simulink model "SimulinkFinal"  (R2023b)
settings: Solver=FixedStepAuto  StartTime=0.0  StopTime=inf  FixedStep=0.01  RelTol=1e-3
StopFcn:
  | % Generate a unique filename based on the current date and time
  | timestamp = datestr(now, 'yyyy-mm-dd_HH-MM-SS');
  | filename = ['simulation_logs_' timestamp '.mat'];
  | 
  | % Check if 'out' variable (SimulationOutput) exists
  | if exist('out', 'var')
  |     % Extract logsout from the simulation output object
  |     logsout = out.logsout;
  | 
  |     % Save the logsout variable to a .mat file
  |     save(filename, 'logsout');
  | else
  |     warning('Simulation output not found. No data saved.');
  | end
model workspace (MAT data in the model file):
  SL_ROS_VariableLengthArrays_MaxSizes.CommonInfo.ArrayTruncateAction = 'EmitWarning'
  SL_ROS_VariableLengthArrays_MaxSizes.MsgTypeMap = containers.Map
  SL_ROS_VariableLengthArrays_MaxSizes.MsgTypeMap.serialization.keys = {'sensor_msgs/Image', 'sensor_msgs/PointCloud2'}
  SL_ROS_VariableLengthArrays_MaxSizes.MsgTypeMap.serialization.values{1}(1).PropertyName = 'data'
  SL_ROS_VariableLengthArrays_MaxSizes.MsgTypeMap.serialization.values{1}(1).DataType = 'uint8'
  SL_ROS_VariableLengthArrays_MaxSizes.MsgTypeMap.serialization.values{1}(1).MaxLength = 1920000
  SL_ROS_VariableLengthArrays_MaxSizes.MsgTypeMap.serialization.values{1}(2).PropertyName = 'encoding'
  SL_ROS_VariableLengthArrays_MaxSizes.MsgTypeMap.serialization.values{1}(2).DataType = 'uint8'
  SL_ROS_VariableLengthArrays_MaxSizes.MsgTypeMap.serialization.values{1}(2).MaxLength = 128
  SL_ROS_VariableLengthArrays_MaxSizes.MsgTypeMap.serialization.values{2}(1).PropertyName = 'data'
  SL_ROS_VariableLengthArrays_MaxSizes.MsgTypeMap.serialization.values{2}(1).DataType = 'uint8'
  SL_ROS_VariableLengthArrays_MaxSizes.MsgTypeMap.serialization.values{2}(1).MaxLength = 390000
  SL_ROS_VariableLengthArrays_MaxSizes.MsgTypeMap.serialization.values{2}(2).PropertyName = 'fields'
  SL_ROS_VariableLengthArrays_MaxSizes.MsgTypeMap.serialization.values{2}(2).DataType = 'sensor_msgs/PointField'
  SL_ROS_VariableLengthArrays_MaxSizes.MsgTypeMap.serialization.values{2}(2).MaxLength = 16
  SL_ROS_VariableLengthArrays_MaxSizes.MsgTypeMap.serialization.uniformity = 0
  SL_ROS_VariableLengthArrays_MaxSizes.MsgTypeMap.serialization.keyType = 'char'
  SL_ROS_VariableLengthArrays_MaxSizes.MsgTypeMap.serialization.valueType = 'any'
undefined symbols (not defined in the file or in its folder): brake, reverse, steer, throttle
libraries: ros2lib x7, slpidlib x1
settings Model: Creator=pruthvi  LastModifiedBy=pruthvi
settings OptimizationCC: EnhancedBackFolding=on  PassReuseOutputArgsAs=Individual arguments  ZeroExternalMemoryAtStartup=off  ZeroInternalMemoryAtStartup=off  MaxStackSize=64  OptimizeBlockOrder=speed  DifferentSizesBufferReuse=on  OptimizationCustomize=off  EfficientTunableParamExpr=on
settings DebuggingCC: ParameterPrecisionLossMsg=none  ParameterTunabilityLossMsg=error
settings HardwareCC: UseEmbeddedCoderFeatures=off
settings SFSimCC: MATLABDynamicMemAlloc=off
settings RTWCC: Description=Embedded Coder  SystemTargetFile=ert.tlc  HardwareBoard=Robot Operating System 2 (ROS 2)  TLCOptions="-aInlineSetEventsForThisBaseRateFcn=TLC_FALSE -aSuppressMultiTaskScheduler=TLC_FALSE  -aRateBasedStepFcn=0"  TemplateMakefile=ert_default_tmf  Toolchain=Colcon Tools  TargetLang=C++
settings CodeAppCC: ForceParamTrailComments=on  IgnoreCustomStorageClasses=off  OperatorAnnotations=on  SimulinkDataObjDesc=on  SFDataObjDesc=on  InsertBlockDesc=on
settings ERTTargetCC: CodeInterfacePackaging=C++ class  SupportNonInlinedSFcns=on  RootIOFormat=Structure reference

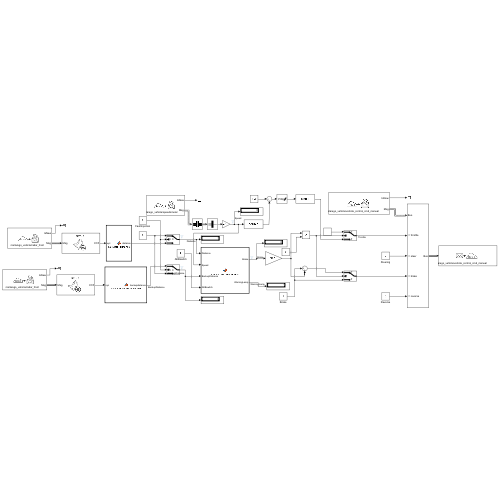
[thumbnail: Simulink's stored preview of the top-level diagram]
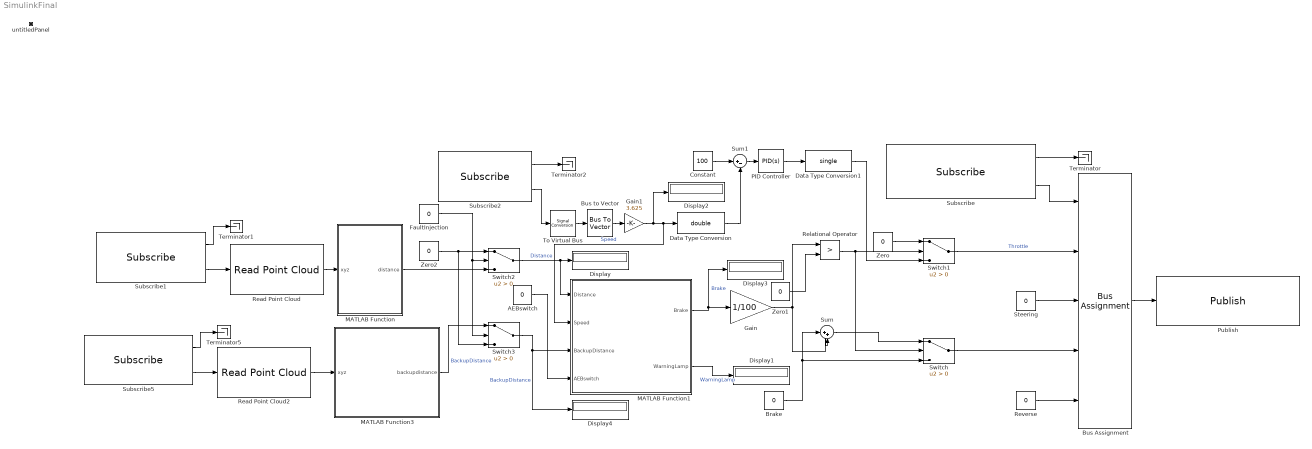
== system SimulinkFinal ==
  AEBswitch : Constant  Value=0  OutDataTypeStr=uint8
  Brake : Constant  Value=0  OutDataTypeStr=single
  Bus Assignment : BusAssignment  AssignedSignals=throttle,steer,brake,reverse
  Bus to Vector : BusToVector
  Constant : Constant  Value=100  OutDataTypeStr=double
  Data Type Conversion : DataTypeConversion  OutDataTypeStr=double  RndMeth=Round  SaturateOnIntegerOverflow=off
  Data Type Conversion1 : DataTypeConversion  OutDataTypeStr=single  RndMeth=Floor
  Display{,1..4} (5 alike) : Display
  FaultInjection : Constant  Value=0
  Gain : Gain  Gain=1/100  OutDataTypeStr=single  RndMeth=Simplest
  Gain1 : Gain  Gain=3.625  OutDataTypeStr=uint8  RndMeth=Round  SaturateOnIntegerOverflow=on
  MATLAB Function : MATLAB Function  TreatAsAtomicUnit=on  SystemSampleTime=0.01
  MATLAB Function1 : MATLAB Function  TreatAsAtomicUnit=on  SystemSampleTime=0.01
  MATLAB Function3 : MATLAB Function  TreatAsAtomicUnit=on  SystemSampleTime=0.01
  PID Controller : slpidlib/PID Controller  Controller=PID  Form=Parallel  TimeDomain=Continuous-time  UseExternalTs=off  SampleTime=-1  IntegratorMethod=Forward Euler  FilterMethod=Forward Euler  ControllerParametersSource=internal  P=0.2  I=0.03  UseKiTs=off  D=0.2  N=100  UseFilter=on  TunerSelectOption=Transfer Function Based (PID Tuner App)  InitialConditionSource=internal  InitialConditionForIntegrator=0  InitialConditionForFilter=0  DifferentiatorICPrevScaledInput=0  ExternalReset=none  TrackingMode=off  Kt=1  LimitOutput=on  SatLimitsSource=internal  UpperSaturationLimit=1  LowerSaturationLimit=0  LinearizeAsGain=on  AntiWindupMode=clamping  Kb=1  LimitIntegrator=on  UpperIntegratorSaturationLimit=1  LowerIntegratorSaturationLimit=0  POutMin=[]  POutMax=[]  IOutMin=[]  IOutMax=[]  DOutMin=[]  DOutMax=[]  NOutMin=[]  NOutMax=[]  SumOutMin=[]  SumOutMax=[]  SaturationOutMin=[]  SaturationOutMax=[]  PParamMin=[]  PParamMax=[]  IParamMin=[]  IParamMax=[]  DParamMin=[]  DParamMax=[]  NParamMin=[]  NParamMax=[]  KbParamMin=[]  KbParamMax=[]  KtParamMin=[]  KtParamMax=[]  KbOutMin=[]  KbOutMax=[]  KtOutMin=[]  KtOutMax=[]  IntegratorOutMin=[]  IntegratorOutMax=[]  FilterOutMin=[]  FilterOutMax=[]  SumI1OutMin=[]  SumI1OutMax=[]  SumI2OutMin=[]  SumI2OutMax=[]  SumI3OutMin=[]  SumI3OutMax=[]  SumI4OutMin=[]  SumI4OutMax=[]  SumDOutMin=[]  SumDOutMax=[]  DifferentiatorOutMin=[]  DifferentiatorOutMax=[]  FilterDiffOutCoefMin=[]  FilterDiffOutCoefMax=[]  ReciprocalOutMin=[]  ReciprocalOutMax=[]  SumDenOutMin=[]  SumDenOutMax=[]  SumNumOutMin=[]  SumNumOutMax=[]  DivideOutMin=[]  DivideOutMax=[]  UdiffTsProdOutMin=[]  UdiffTsProdOutMax=[]  NTsProdOutMin=[]  NTsProdOutMax=[]  UintegralTsProdOutMin=[]  UintegralTsProdOutMax=[]  UngainTsProdOutMin=[]  UngainTsProdOutMax=[]  ClampingZeroOutDataTypeStr=Inherit: Inherit via back propagation  ClampingZeroOutMin=[]  ClampingZeroOutMax=[]  FilterDenConstantOutDataTypeStr=Inherit: Inherit via back propagation  FilterDenConstantOutMin=[]  FilterDenConstantOutMax=[]  PCopyOutDataTypeStr=Inherit: Inherit via back propagation  PCopyOutMin=[]  PCopyOutMax=[]  NCopyOutDataTypeStr=Inherit: Inherit via back propagation  NCopyOutMin=[]  NCopyOutMax=[]  IntegratorContinuousStateAttributes=''  IntegratorStateMustResolveToSignalObject=off  IntegratorRTWStateStorageClass=Auto  FilterContinuousStateAttributes=''  FilterStateMustResolveToSignalObject=off  FilterRTWStateStorageClass=Auto  ParallelPVariant=InternalParameters  IdealPVariant=Disabled  IVariant=InternalParameters  DVariant=InternalParameters  IntegratorVariant=Continuous  SatVariant=Enabled  AWVariant=ContClampingParallel  PCopyVariant=Disabled  TRVariant=Disabled  FdbkBlocksVariant=Forward  IdealPFdbkVariant=Disabled  SatFdbkVariant=Disabled  DerivativeFilterVariant=ContFilter  NVariant=InternalParameters  NCopyVariant=Disabled  FilterICVariant=InternalICsFilter  IntegratorICVariant=InternalICs  ExternalResetVariant=Disabled  TRSumVariant=Passthrough  SumFdbkVariant=Disabled  SumVariant=Sum_PID  TsampFilterVariant=InternalTs  TsampNgainVariant=Passthrough  TsampIntegralVariant=Disabled_SignalSpec  ExternalSaturationOutDataTypeStr=Inherit: Same as second input
  Publish : ros2lib/Publish  topicSource=Select from ROS network  topic=/carla/ego_vehicle/vehicle_control_cmd_manual  messageType=carla_msgs/CarlaEgoVehicleControl  QOSHistory=Keep last  QOSDepth=1  QOSReliability=Reliable  QOSDurability=Volatile
  Read Point Cloud : ros2lib/Read Point Cloud  MaximumPointCloudSize=[1, 8254]  PreserveStructure=off  ShowRGBOutput=off  ShowIntensityOutput=off  ShowErrorCodeOutput=off  VariableSizeOutputs=off
  Read Point Cloud2 : ros2lib/Read Point Cloud  MaximumPointCloudSize=[1, 8254]  PreserveStructure=off  ShowRGBOutput=off  ShowIntensityOutput=off  ShowErrorCodeOutput=off  VariableSizeOutputs=off
  Relational Operator : RelationalOperator  Operator=>  OutDataTypeStr=boolean  RndMeth=Simplest  InputSameDT=off
  Reverse : Constant  Value=0  OutDataTypeStr=boolean
  Steering : Constant  Value=0  OutDataTypeStr=single
  Subscribe : ros2lib/Subscribe  topicSource=Select from ROS network  topic=/carla/ego_vehicle/vehicle_control_cmd_manual  messageType=carla_msgs/CarlaEgoVehicleControl  sampleTime=-1  QOSHistory=Keep last  QOSDepth=1  QOSReliability=Reliable  QOSDurability=Volatile
  Subscribe1 : ros2lib/Subscribe  topicSource=Select from ROS network  topic=/carla/ego_vehicle/radar_front  messageType=sensor_msgs/PointCloud2  sampleTime=0.2  QOSHistory=Keep last  QOSDepth=1  QOSReliability=Reliable  QOSDurability=Volatile
  Subscribe2 : ros2lib/Subscribe  topicSource=Select from ROS network  topic=/carla/ego_vehicle/speedometer  messageType=std_msgs/Float32  sampleTime=-1  QOSHistory=Keep last  QOSDepth=1  QOSReliability=Reliable  QOSDurability=Volatile
  Subscribe5 : ros2lib/Subscribe  topicSource=Select from ROS network  topic=/carla/ego_vehicle/radar_front  messageType=sensor_msgs/PointCloud2  sampleTime=0.2  QOSHistory=Keep last  QOSDepth=1  QOSReliability=Reliable  QOSDurability=Volatile
  Sum : Sum  Inputs=|++
  Sum1 : Sum  Inputs=|+-
  Switch{,1..3} (4 alike) : Switch  Criteria=u2 > Threshold  SaturateOnIntegerOverflow=off  InputSameDT=off
  Terminator{,1..2,5} (4 alike) : Terminator
  To Virtual Bus : SignalConversion  ConversionOutput=Virtual bus  OverrideOpt=off
  Zero : Constant  Value=0  OutDataTypeStr=Inherit: Inherit via back propagation
  Zero1 : Constant  Value=0  OutDataTypeStr=Inherit: Inherit via back propagation
  Zero2 : Constant  Value=0  OutDataTypeStr=Inherit: Inherit via back propagation
  untitledPanel : Subsystem  Tag=HiddenForWebPanel  IsWebBlockPanel=on
  wires:
  Subscribe2/1 -> Terminator2/1
  Subscribe5/1 -> Terminator5/1
  Constant/1 -> Sum1/1
  Subscribe1/2 -> Read Point Cloud/1
  Data Type Conversion1/1 -> Switch1/3
  To Virtual Bus/1 -> Bus to Vector/1
  Subscribe1/1 -> Terminator1/1
  Zero/1 -> Switch1/1
  Subscribe2/2 -> To Virtual Bus/1
  MATLAB Function/1(distance) -> Switch2/3
  Bus to Vector/1 -> Gain1/1
  Data Type Conversion/1 -> Sum1/2
  Subscribe5/2 -> Read Point Cloud2/1
  Read Point Cloud/1 -> MATLAB Function/1(xyz)
  Zero1/1 -> Relational Operator/2
  Read Point Cloud2/1 -> MATLAB Function3/1(xyz)
  Reverse/1 -> Bus Assignment/5
  Gain1/1 -> Display2/1, MATLAB Function1/2(Speed), Data Type Conversion/1  "Speed"
  Sum1/1 -> PID Controller/1
  FaultInjection/1 -> Switch3/2, Switch2/2
  Steering/1 -> Bus Assignment/3
  Zero2/1 -> Switch2/1, Switch3/3
  MATLAB Function3/1(backupdistance) -> Switch3/1  "BackupDistance"
  Switch2/1 -> MATLAB Function1/1(Distance), Display/1  "Distance"
  MATLAB Function1/1(Brake) -> Display3/1, Gain/1  "Brake"
  AEBswitch/1 -> MATLAB Function1/4(AEBswitch)
  PID Controller/1 -> Data Type Conversion1/1
  Switch3/1 -> MATLAB Function1/3(BackupDistance), Display4/1  "BackupDistance"
  Switch1/1 -> Bus Assignment/2  "Throttle"
  Relational Operator/1 -> Switch/2, Switch1/2
  MATLAB Function1/2(WarningLamp) -> Display1/1  "WarningLamp"
  Gain/1 -> Sum/2, Relational Operator/1
  Brake/1 -> Sum/1, Switch/3
  Sum/1 -> Switch/1
  Subscribe/1 -> Terminator/1
  Subscribe/2 -> Bus Assignment/1
  Switch/1 -> Bus Assignment/4
  Bus Assignment/1 -> Publish/1

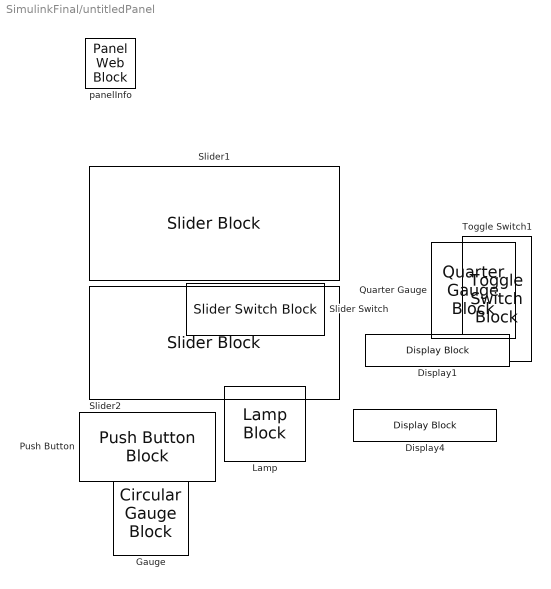
== system SimulinkFinal/untitledPanel ==
  Display1 : DisplayBlock  Tag=HiddenForWebPanel  PanelInfo="{\"addnFilesFolder\":\"\",\"height\":59,\"includeDebugPackages\":false,\"left\":281,\"outputFolder\":\"\",\"panelId\":\"panelId-4ec24f18-4b2b-4da9-8655-6245c59e87f1\",\"popoutMode\":\"\",\"standaloneTitle\":\"\",\"top\":316,\"type\":\"panelChild\",\"version\":\"2019b\",\"width\":174,\"zIndex\":1500038}"  Transparency=1
  Display4 : DisplayBlock  Tag=HiddenForWebPanel  PanelInfo="{\"addnFilesFolder\":\"\",\"height\":60,\"includeDebugPackages\":false,\"left\":283,\"outputFolder\":\"\",\"panelId\":\"panelId-4ec24f18-4b2b-4da9-8655-6245c59e87f1\",\"popoutMode\":\"\",\"standaloneTitle\":\"\",\"top\":386,\"type\":\"panelChild\",\"version\":\"2019b\",\"width\":169,\"zIndex\":1500040}"  Transparency=1
  Gauge : CircularGaugeBlock  Tag=HiddenForWebPanel  PanelInfo="{\"addnFilesFolder\":\"\",\"height\":153,\"includeDebugPackages\":false,\"left\":274,\"outputFolder\":\"\",\"panelId\":\"panelId-4ec24f18-4b2b-4da9-8655-6245c59e87f1\",\"popoutMode\":\"\",\"standaloneTitle\":\"\",\"top\":23,\"type\":\"panelChild\",\"version\":\"2019b\",\"width\":194,\"zIndex\":1500022}"  TickInterval=10
  Lamp : LampBlock  Tag=HiddenForWebPanel  PanelInfo="{\"addnFilesFolder\":\"\",\"height\":65,\"includeDebugPackages\":false,\"left\":178,\"outputFolder\":\"\",\"panelId\":\"panelId-4ec24f18-4b2b-4da9-8655-6245c59e87f1\",\"popoutMode\":\"\",\"standaloneTitle\":\"\",\"top\":365,\"type\":\"panelChild\",\"version\":\"2019b\",\"width\":96,\"zIndex\":1500042}"
  Push Button : PushButtonBlock  Tag=HiddenForWebPanel  PanelInfo="{\"addnFilesFolder\":\"\",\"height\":87,\"includeDebugPackages\":false,\"left\":19,\"outputFolder\":\"\",\"panelId\":\"panelId-4ec24f18-4b2b-4da9-8655-6245c59e87f1\",\"popoutMode\":\"\",\"standaloneTitle\":\"\",\"top\":361,\"type\":\"panelChild\",\"version\":\"2019b\",\"width\":151,\"zIndex\":1500044}"  LabelPosition=Top  ButtonText=SensorFailure  ButtonType=Latch  Icon=CheckEngine2  IconColor=On  OffValue=0.000000
  Quarter Gauge : QuarterGaugeBlock  Tag=HiddenForWebPanel  PanelInfo="{\"addnFilesFolder\":\"\",\"height\":121,\"includeDebugPackages\":false,\"left\":283,\"outputFolder\":\"\",\"panelId\":\"panelId-4ec24f18-4b2b-4da9-8655-6245c59e87f1\",\"popoutMode\":\"\",\"standaloneTitle\":\"\",\"top\":183,\"type\":\"panelChild\",\"version\":\"2019b\",\"width\":168,\"zIndex\":1500024}"  TickInterval=25
  Slider Switch : SliderSwitchBlock  Tag=HiddenForWebPanel  PanelInfo="{\"addnFilesFolder\":\"\",\"height\":54,\"includeDebugPackages\":false,\"left\":105,\"outputFolder\":\"\",\"panelId\":\"panelId-4ec24f18-4b2b-4da9-8655-6245c59e87f1\",\"popoutMode\":\"\",\"standaloneTitle\":\"\",\"top\":268,\"type\":\"panelChild\",\"version\":\"2019b\",\"width\":146,\"zIndex\":1500036}"
      settings: Values={{'Off', 'On'}, [0 1]}
  Slider1 : SliderBlock  Tag=HiddenForWebPanel  PanelInfo="{\"addnFilesFolder\":\"\",\"height\":114,\"includeDebugPackages\":false,\"left\":15,\"outputFolder\":\"\",\"panelId\":\"panelId-4ec24f18-4b2b-4da9-8655-6245c59e87f1\",\"popoutMode\":\"\",\"standaloneTitle\":\"\",\"top\":18,\"type\":\"panelChild\",\"version\":\"2019b\",\"width\":250,\"zIndex\":1500018}"  ScaleMin=-1  ScaleMax=1  TickInterval=1
  Slider2 : SliderBlock  Tag=HiddenForWebPanel  PanelInfo="{\"addnFilesFolder\":\"\",\"height\":113,\"includeDebugPackages\":false,\"left\":15,\"outputFolder\":\"\",\"panelId\":\"panelId-4ec24f18-4b2b-4da9-8655-6245c59e87f1\",\"popoutMode\":\"\",\"standaloneTitle\":\"\",\"top\":138,\"type\":\"panelChild\",\"version\":\"2019b\",\"width\":250,\"zIndex\":1500010}"  ScaleMax=1  TickInterval=0.5
  Toggle Switch1 : ToggleSwitchBlock  Tag=HiddenForWebPanel  PanelInfo="{\"addnFilesFolder\":\"\",\"height\":96,\"includeDebugPackages\":false,\"left\":19,\"outputFolder\":\"\",\"panelId\":\"panelId-4ec24f18-4b2b-4da9-8655-6245c59e87f1\",\"popoutMode\":\"\",\"standaloneTitle\":\"\",\"top\":258,\"type\":\"panelChild\",\"version\":\"2019b\",\"width\":50,\"zIndex\":1500008}"
      settings: Values={{'Off', 'On'}, [0 1]}
  panelInfo : PanelWebBlock  Tag=HiddenForWebPanel  PanelInfo="{\"addnFilesFolder\":\"\",\"compacted\":false,\"height\":465,\"includeDebugPackages\":false,\"isActiveTab\":true,\"left\":17,\"name\":\"Panel\",\"outputFolder\":\"\",\"panelId\":\"panelId-4ec24f18-4b2b-4da9-8655-6245c59e87f1\",\"popoutMode\":\"\",\"standaloneTitle\":\"\",\"tabIndex\":0,\"tabbedSetId\":\"tabbedSet3834338684\",\"top\":33,\"type\":\"panel\",\"version\":\"2019b\",\"visible\":true,\"width\":474,\"zIndex\":1500002}"

== matlab function SimulinkFinal/MATLAB Function1 ==
  data: Distance input; Speed input; BackupDistance input; AEBswitch input; Brake output; WarningLamp output
function [Brake, WarningLamp] = emergencyBrakingLogic(Distance, Speed, BackupDistance, AEBswitch)
% EMERGENCYBRAKINGLOGIC Calculate brake intensity based on filtered distance
% Distance: Smoothed distance data (single)
% Speed: Vehicle speed in kmph (uint8)
% BackupDistance: Backup distance input in case primary fails (uint8)
% AEBswitch: Automatic Emergency Braking switch (1 for ON, 0 for OFF)
% Brake: Braking intensity as a value from 0 to 100 (uint8)
% WarningLamp: Warning signal output (1 if primary sensor fails, 0 otherwise)

persistent brake_history brake_active threshold_set Distance_threshold min_distance;
window_size = 300; % Larger window size for even smoother results (adjustable)

% Initialize persistent variables
if isempty(brake_history)
    brake_history = single(zeros(window_size, 1));
    brake_active = false; % Flag to indicate if brake should stay fully on
    threshold_set = false; % Flag to check if threshold has been set based on initial distance check
    Distance_threshold = single(20); % Default threshold to 20 if speed <= 55
    min_distance = single(12); % Minimum distance for full braking application
end

% Initialize output values
Brake = uint8(0);
WarningLamp = uint8(0); % Default to 0, indicating no warning

% Convert Distance and BackupDistance from uint8 to single for calculations
Distance = single(Distance);
BackupDistance = single(BackupDistance);
max_Brake = single(100); % Maximum brake intensity (0 to 100)

% Check if primary Distance data is valid (non-zero and received)
if Distance <= 0
    % If primary distance is invalid, switch to backup and activate warning
    Distance = BackupDistance;
    WarningLamp = uint8(1); % Set warning signal to 1
end

% Reset brake if AEB is switched off
if AEBswitch == 0
    brake_active = false; % Reset the brake active flag when AEB is off
    Brake = uint8(0); % No brake when AEB is off
    WarningLamp = uint8(1); % Set warning signal to 1
    threshold_set = false; % Reset threshold check
    Distance_threshold = single(20); % Reset to default threshold
    min_distance = single(12); % Reset to default minimum distance
    return;
end

% Check distance and set threshold based on speed when distance drops below 22 for the first time
if Distance < 22 && ~threshold_set
    if Speed > 55
        Distance_threshold = single(22); % Set threshold to 22 if speed > 55
        min_distance = single(20); % Set minimum distance to 20 if speed > 55
    else
        Distance_threshold = single(20); % Set threshold to 20 if speed <= 55
        min_distance = single(12); % Set minimum distance to 12 if speed <= 55
    end
    threshold_set = true; % Threshold set, so do not reset
end

% Braking logic
% Once the distance is below min_distance, brake remains fully engaged
if Distance <= min_distance && Speed > 10
    brake_active = true; % Activate the brake persistence when distance is below min_distance
end

% If the brake is active, keep it fully engaged
if brake_active
    Brake = uint8(100); % Keep brake fully applied
    return; % No further calculations needed
end

% Normal braking logic before the distance drops below min_distance
if AEBswitch == 1
    if Distance <= Distance_threshold && Distance > min_distance
        % Linear braking response for smoother braking
        Brake_value = max_Brake * (Distance_threshold - Distance) / (Distance_threshold - min_distance);
    elseif Distance <= min_distance
        Brake_value = max_Brake;
    else
        Brake_value = single(0);
    end
    
    Brake = uint8(round(Brake_value));
end
end

== matlab function SimulinkFinal/MATLAB Function ==
  data: xyz input; distance output
function distance = calculate_distance(xyz)
% CALCULATE_distance Calculate the minimum distance of objects in front of the vehicle
% xyz: Radar point cloud data [N x 3] where each row is (x, y, z)
% distance: minimum distance to an object in front of the vehicle in meters (single)

% Define parameters
vehicle_width = single(2); % Vehicle width (meters)

% Initialize persistent variable to store locked distance
persistent locked_distance;

% Set initial distance to 0
distance = uint8(0);

% Ensure there are points to process
if isempty(xyz)
    return; % Return 0 if no points are available
end

% Filter points within the specified lateral range (front of the vehicle)
front_indices = abs(single(xyz(:, 2))) <= vehicle_width;

% Ensure there are points in the front
if ~any(front_indices)
    return; % Return 0 if no points are detected in the front
end

% Filtered points
front_points = single(xyz(front_indices, :));

% Calculate distances of the filtered points from the origin (vehicle position)
distances = sqrt(sum(front_points.^2, 2));

% Ensure there are valid distances
if isempty(distances)
    return; % Return 0 if no valid distances are found
end

% Find the minimum distance
current_min_distance = min(distances);

% If locked_distance is empty, initialize it with the current minimum distance
if isempty(locked_distance)
    locked_distance = current_min_distance;
end

% If the distance goes below 7, lock it at that value
if current_min_distance < 7
    locked_distance = min(locked_distance, 7);
else
    % Update locked_distance if the minimum distance hasn't gone below 7
    locked_distance = min(locked_distance, current_min_distance);
end

% Return the locked distance as uint8
distance = uint8(round(locked_distance));
end

== matlab function SimulinkFinal/MATLAB Function3 ==
  data: xyz input; backupdistance output
function backupdistance = calculate_backupdistance(xyz)
% CALCULATE_backupdistance Calculate the minimum backupdistance of objects in front of the vehicle
% xyz: Radar point cloud data [N x 3] where each row is (x, y, z)
% backupdistance: minimum backupdistance to an object in front of the vehicle in meters (single)

% Define parameters
vehicle_width = single(2); % Vehicle width (meters)

% Initialize persistent variable to store locked backupdistance
persistent locked_backupdistance;

% Set initial backupdistance to 0
backupdistance = uint8(0);

% Ensure there are points to process
if isempty(xyz)
    return; % Return 0 if no points are available
end

% Filter points within the specified lateral range (front of the vehicle)
front_indices = abs(single(xyz(:, 2))) <= vehicle_width;

% Ensure there are points in the front
if ~any(front_indices)
    return; % Return 0 if no points are detected in the front
end

% Filtered points
front_points = single(xyz(front_indices, :));

% Calculate backupdistances of the filtered points from the origin (vehicle position)
backupdistances = sqrt(sum(front_points.^2, 2));

% Ensure there are valid backupdistances
if isempty(backupdistances)
    return; % Return 0 if no valid backupdistances are found
end

% Find the minimum backupdistance
current_min_distance = min(backupdistances);

% If locked_backupdistance is empty, initialize it with the current minimum distance
if isempty(locked_backupdistance)
    locked_backupdistance = current_min_distance;
end

% If the distance goes below 7, lock it at that value
if current_min_distance < 7
    locked_backupdistance = min(locked_backupdistance, 7);
else
    % Update locked_backupdistance if the minimum distance hasn't gone below 7
    locked_backupdistance = min(locked_backupdistance, current_min_distance);
end

% Return the locked backupdistance as uint8
backupdistance = uint8(round(locked_backupdistance));
end
